simulink model "car_model"  (R2017a)
settings: Solver=VariableStepAuto  StartTime=0.0  StopTime=tf  RelTol=1e-3  AbsTol=1e-6
values from neighbouring files (symbols this model uses):
  MAX_DELTA_i = deg2rad(MAX_DELTA_i)    [run_sim.m]
  x0 = double(subs([qs0; ps0], symbs, vals))    [run_sim.m]
undefined symbols (not defined in the file or in its folder): sys
(part 1 of 2)
settings Model: Creator=brunolnetto  LastModifiedBy=brunolnetto
settings DataIOCC: SaveState=on  StateSaveName=xoutNew  OutputSaveName=youtNew

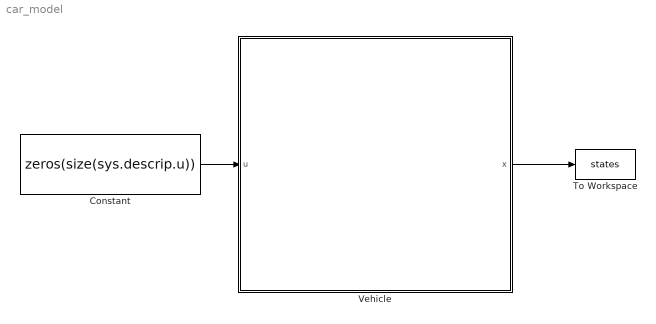
== system car_model ==
  Constant : Constant  Value=zeros(size(sys.descrip.u))
  To Workspace : ToWorkspace  VariableName=states  SaveFormat=Structure With Time  SampleTime=-1
  Vehicle : Subsystem
      mask Display: image('/home/brunolnetto/Pictures/auto_model.png');
  wires:
  Constant/1 -> Vehicle/1(u)
  Vehicle/1(x) -> To Workspace/1

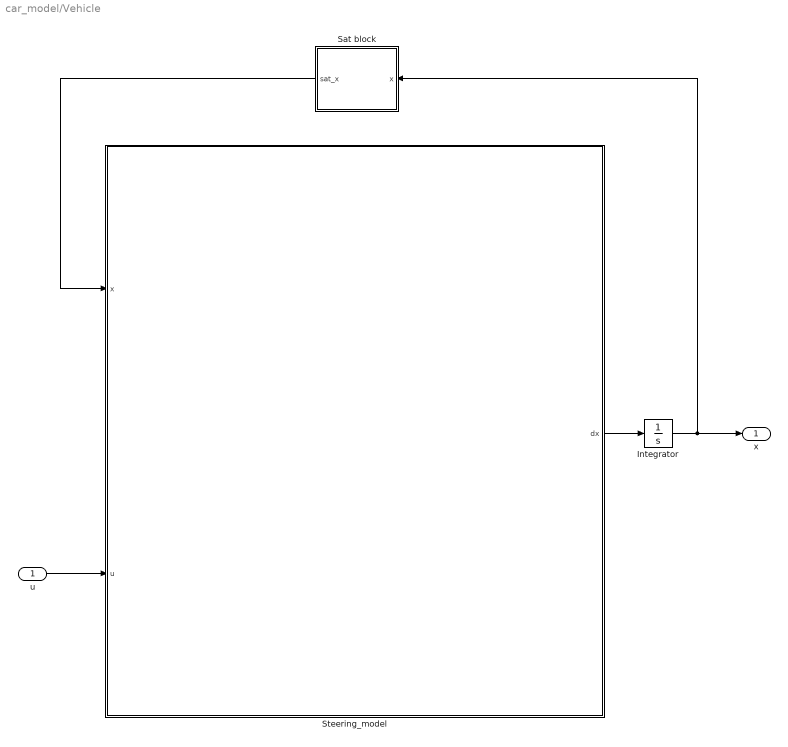
== system car_model/Vehicle ==
  u : Inport
  Integrator : Integrator  InitialCondition=x0
  Sat block : Subsystem
  Steering_model : Subsystem
      mask Display: image('/home/brunolnetto/Pictures/steer_schema.png');
  x : Outport
  wires:
  Steering_model/1(dx) -> Integrator/1
  u/1 -> Steering_model/2(u)
  Integrator/1 -> x/1, Sat block/1(x)
  Sat block/1(sat_x) -> Steering_model/1(x)

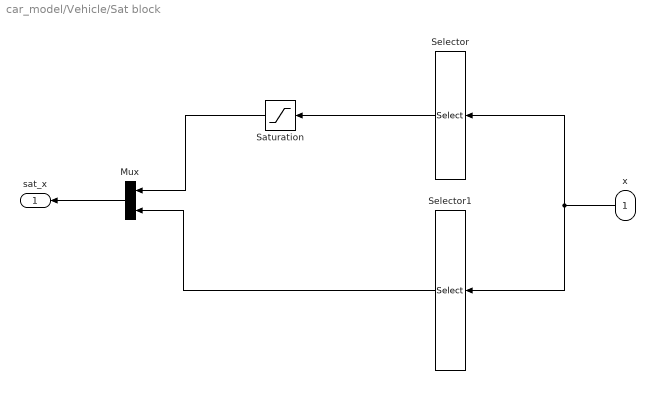
== system car_model/Vehicle/Sat block ==
  x : Inport
  Mux : Mux  Inputs=2
  Saturation : Saturate  UpperLimit=MAX_DELTA_i  LowerLimit=-MAX_DELTA_i
  Selector : Selector  InputPortWidth=13  IndexOptions=Index vector (dialog)  Indices=4  OutputSizes=1
  Selector1 : Selector  InputPortWidth=13  IndexOptions=Index vector (dialog)  Indices=[1 2. 3. 5. 6. 7. 8. 9. 10. 11. 12. 13]  OutputSizes=1
  sat_x : Outport
  wires:
  Saturation/1 -> Mux/1
  Selector/1 -> Saturation/1
  Mux/1 -> sat_x/1
  x/1 -> Selector1/1, Selector/1
  Selector1/1 -> Mux/2

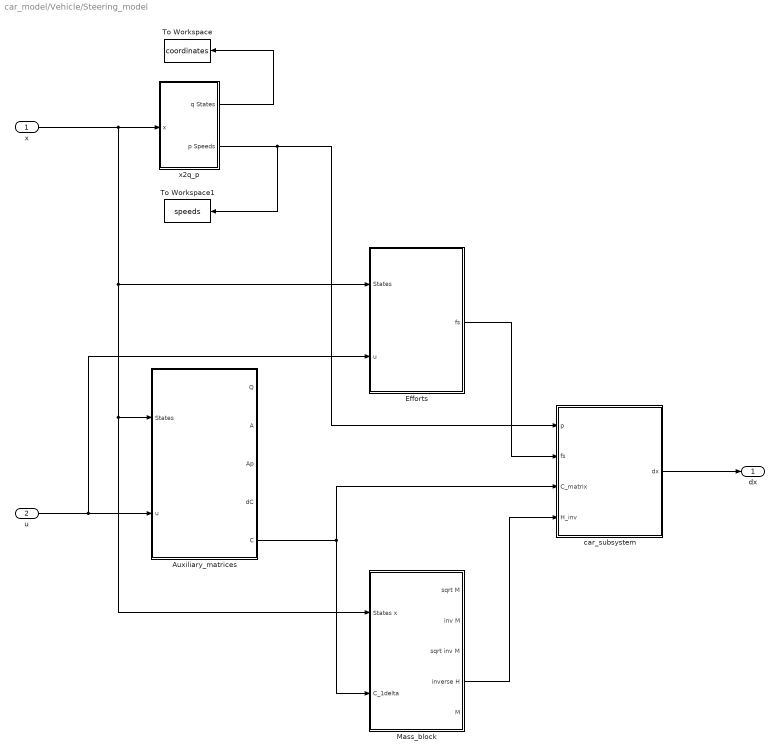
== system car_model/Vehicle/Steering_model ==
  x : Inport
  u : Inport  Port=2
  Auxiliary_matrices : Subsystem
  Efforts : Subsystem
  Mass_block : Subsystem
  To Workspace : ToWorkspace  VariableName=coordinates  SaveFormat=Structure With Time  SampleTime=-1
  To Workspace1 : ToWorkspace  VariableName=speeds  SaveFormat=Structure With Time  SampleTime=-1
  car_subsystem : Subsystem
  x2q_p : Subsystem
  dx : Outport
  wires:
  Auxiliary_matrices/5(C) -> car_subsystem/3(C_matrix), Mass_block/2("C_1delta  ")
  u/1 -> Efforts/2(u), Auxiliary_matrices/2(u)
  Mass_block/4(inverse H) -> car_subsystem/4(H_inv)
  car_subsystem/1(dx) -> dx/1
  Efforts/1(fs) -> car_subsystem/2(fs)
  x2q_p/1(q States) -> To Workspace/1
  x2q_p/2(p Speeds) -> To Workspace1/1, car_subsystem/1(p)
  x/1 -> x2q_p/1(x), Efforts/1(States), Mass_block/1(States x), Auxiliary_matrices/1(States)

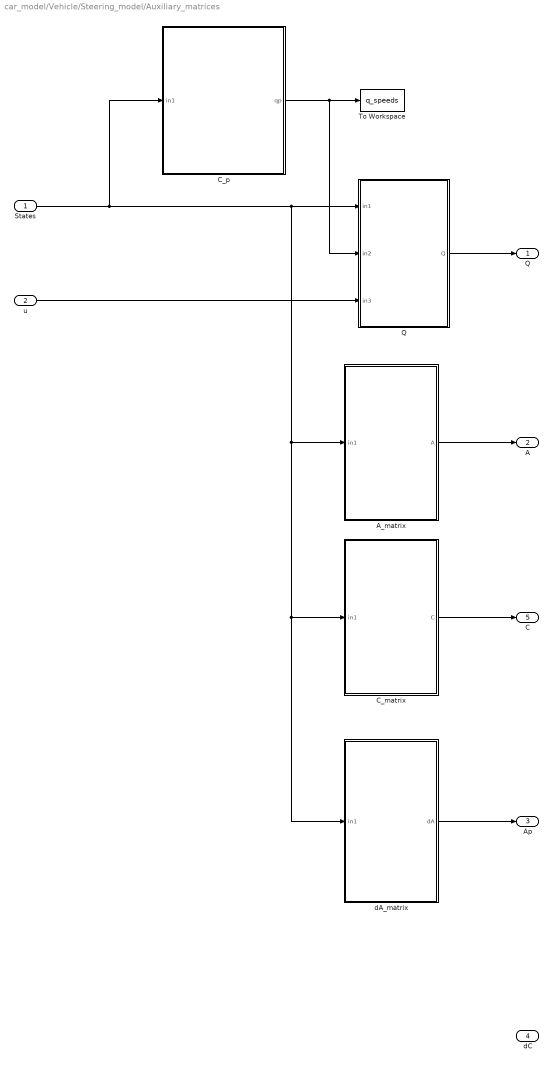
== system car_model/Vehicle/Steering_model/Auxiliary_matrices ==
  States : Inport
  u : Inport  Port=2
  A_matrix : MATLAB Function  TreatAsAtomicUnit=on
  C_matrix : MATLAB Function  TreatAsAtomicUnit=on
  C_p : MATLAB Function  TreatAsAtomicUnit=on
  Q : MATLAB Function  TreatAsAtomicUnit=on
  To Workspace : ToWorkspace  VariableName=q_speeds  SaveFormat=Structure With Time  SampleTime=-1
  dA_matrix : MATLAB Function  TreatAsAtomicUnit=on
  "Q " : Outport
  A : Outport  Port=2
  Ap : Outport  Port=3
  dC : Outport  Port=4
  C : Outport  Port=5
  wires:
  C_matrix/1(C) -> C/1
  Q/1(Q) -> "Q "/1
  A_matrix/1(A) -> A/1
  dA_matrix/1(dA) -> Ap/1
  u/1 -> Q/3(in3)
  States/1 -> C_p/1(in1), dA_matrix/1(in1), C_matrix/1(in1), A_matrix/1(in1), Q/1(in1)
  C_p/1(qp) -> To Workspace/1, Q/2(in2)

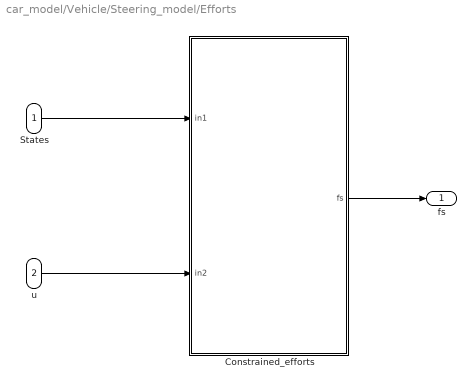
== system car_model/Vehicle/Steering_model/Efforts ==
  States : Inport
  u : Inport  Port=2
  Constrained_efforts : MATLAB Function  TreatAsAtomicUnit=on
  fs : Outport
  wires:
  States/1 -> Constrained_efforts/1(in1)
  u/1 -> Constrained_efforts/2(in2)
  Constrained_efforts/1(fs) -> fs/1

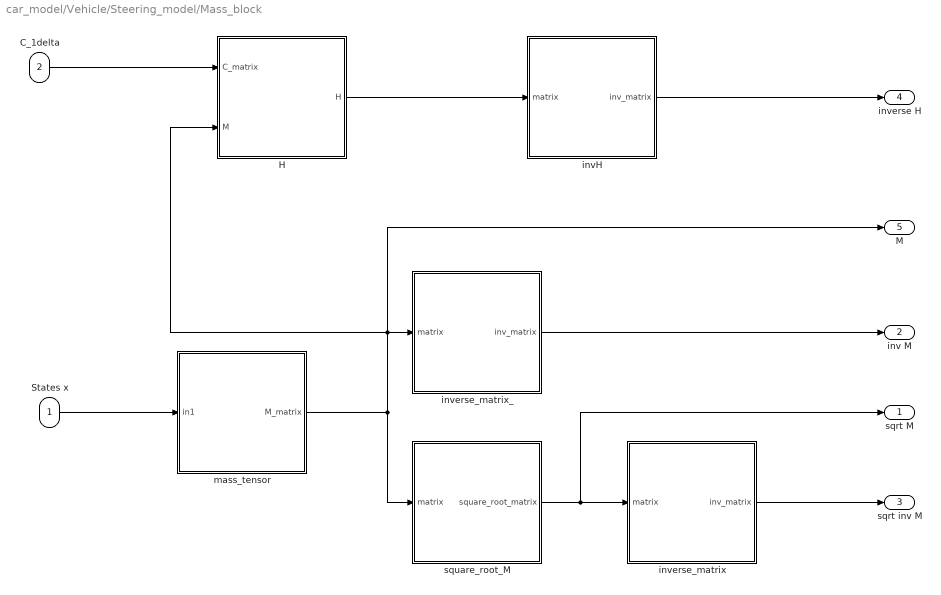
== system car_model/Vehicle/Steering_model/Mass_block ==
  States x : Inport
  "C_1delta  " : Inport  Port=2
  H : MATLAB Function  TreatAsAtomicUnit=on
  invH : MATLAB Function  TreatAsAtomicUnit=on
  inverse_matrix : MATLAB Function  TreatAsAtomicUnit=on
  inverse_matrix_ : MATLAB Function  TreatAsAtomicUnit=on
  mass_tensor : MATLAB Function  TreatAsAtomicUnit=on
  square_root_M : MATLAB Function  TreatAsAtomicUnit=on
  sqrt M : Outport
  inv M : Outport  Port=2
  sqrt inv M : Outport  Port=3
  inverse H : Outport  Port=4
  M : Outport  Port=5
  wires:
  States x/1 -> mass_tensor/1(in1)
  "C_1delta  "/1 -> H/1(C_matrix)
  inverse_matrix_/1(inv_matrix) -> inv M/1
  H/1(H) -> invH/1(matrix)
  invH/1(inv_matrix) -> inverse H/1
  inverse_matrix/1(inv_matrix) -> sqrt inv M/1
  mass_tensor/1(M_matrix) -> M/1, H/2(M), inverse_matrix_/1(matrix), square_root_M/1(matrix)
  square_root_M/1(square_root_matrix) -> sqrt M/1, inverse_matrix/1(matrix)

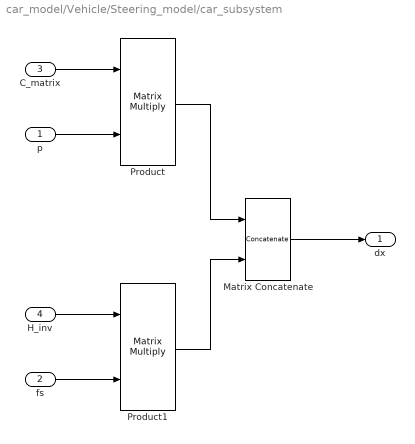
== system car_model/Vehicle/Steering_model/car_subsystem ==
  p : Inport
  fs : Inport  Port=2
  C_matrix : Inport  Port=3
  H_inv : Inport  Port=4
  Matrix Concatenate : Concatenate  ConcatenateDimension=2
  Product : Product  Multiplication=Matrix(*)
  Product1 : Product  Multiplication=Matrix(*)
  dx : Outport
  wires:
  Product/1 -> Matrix Concatenate/1
  p/1 -> Product/2
  C_matrix/1 -> Product/1
  Product1/1 -> Matrix Concatenate/2
  H_inv/1 -> Product1/1
  fs/1 -> Product1/2
  Matrix Concatenate/1 -> dx/1

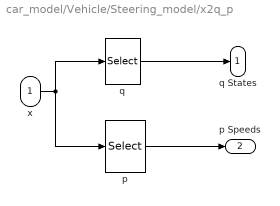
== system car_model/Vehicle/Steering_model/x2q_p ==
  x : Inport
  p : Selector  InputPortWidth=13  IndexOptions=Index vector (dialog)  Indices=[10 11 12 13]  OutputSizes=1
  q : Selector  InputPortWidth=13  IndexOptions=Index vector (dialog)  Indices=[1 2 3 4 5 6 7 8 9]  OutputSizes=1
  q States : Outport
  p Speeds : Outport  Port=2
  wires:
  x/1 -> p/1, q/1
  q/1 -> q States/1
  p/1 -> p Speeds/1

== matlab function car_model/Vehicle/Steering_model/Auxiliary_matrices/A_matrix ==
  data: in1 input; A output
function A = ConstraintMatrix(in1)

%    This function was generated by the Symbolic Math Toolbox version 7.2.

%    28-Oct-2020 21:52:18



delta_i = in1(4,:);

delta_o = in1(5,:);

theta = in1(3,:);

t2 = tan(delta_i);

t3 = tan(delta_o);

t4 = t2.*(3.0./2.0);

t5 = delta_i+theta;

t6 = cos(delta_i);

t7 = sin(t5);

t8 = cos(t5);

t9 = sin(delta_i);

A = reshape([0.0,0.0,0.0,t8,-t7,0.0,0.0,0.0,t7,t8,0.0,0.0,0.0,t6.*(-9.0./2.0)+t9.*(3.0./4.0),t6.*(3.0./4.0)+t9.*(9.0./2.0),(t3.*(3.0./2.0)-9.0./2.0).*(t2.^2+1.0).*(-2.0./9.0),0.0,0.0,0.0,0.0,(t3.^2+1.0).*(t4+9.0./2.0).*(-2.0./9.0),0.0,0.0,0.0,0.0,0.0,0.0,1.0./t6,-3.442462000000001e-1,0.0,0.0,0.0,(t4-9.0)./(cos(delta_o).*(t4+9.0)),0.0,0.0,0.0,t2.*(-1.0./3.0)-1.0,0.0,0.0,0.0,0.0,1.0,0.0,0.0,0.0],[5,9]);

end

== matlab function car_model/Vehicle/Steering_model/Mass_block/mass_tensor ==
  data: in1 input; M_matrix output
function M_matrix = Mass_matrix(in1)

%    This function was generated by the Symbolic Math Toolbox version 7.2.

%    28-Oct-2020 21:52:21



delta_i = in1(4,:);

delta_o = in1(5,:);

phi_i = in1(6,:);

phi_l = in1(9,:);

phi_o = in1(7,:);

phi_r = in1(8,:);

theta = in1(3,:);

t2 = cos(theta);

t3 = sin(theta);

t4 = cos(phi_i);

t5 = t4.^2;

t6 = cos(phi_l);

t7 = t6.^2;

t8 = cos(phi_o);

t9 = t8.^2;

t10 = cos(phi_r);

t11 = t10.^2;

t12 = t2.^2;

t13 = sin(phi_l);

t14 = t13.^2;

t15 = sin(phi_r);

t16 = t15.^2;

t17 = t3.^2;

t18 = cos(delta_i);

t19 = sin(phi_i);

t20 = t19.^2;

t21 = cos(delta_o);

t22 = sin(phi_o);

t23 = t22.^2;

t24 = t18.^2;

t25 = sin(delta_i);

t26 = t21.^2;

t27 = sin(delta_o);

t28 = t25.^2;

t29 = t20.^2;

t30 = t27.^2;

t31 = t23.^2;

t32 = phi_i.*4.0;

t33 = cos(t32);

t34 = t5.^2;

t35 = t34.*4.147690617505401e-1;

t36 = t12.*t24.*t29.*4.147690617505401e-1;

t37 = t17.*t20.*t24.*2.073845308752701e-1;

t38 = t12.*t20.*t28.*2.073845308752701e-1;

t39 = t17.*t28.*t29.*4.147690617505401e-1;

t40 = t5.*t12.*t20.*t24.*2.073845308752701e-1;

t41 = t5.*t17.*t20.*t28.*2.073845308752701e-1;

t42 = t3.*t5.*t20.*t25.*4.147690617505401e-1;

t43 = t2.*t3.*t18.*t20.*t25.*4.147690617505401e-1;

t44 = phi_o.*4.0;

t45 = cos(t44);

t46 = t9.^2;

t47 = t46.*4.147690617505401e-1;

t48 = t12.*t26.*t31.*4.147690617505401e-1;

t49 = t17.*t23.*t26.*2.073845308752701e-1;

t50 = t12.*t23.*t30.*2.073845308752701e-1;

t51 = t17.*t30.*t31.*4.147690617505401e-1;

t52 = t9.*t12.*t23.*t26.*2.073845308752701e-1;

t53 = t9.*t17.*t23.*t30.*2.073845308752701e-1;

t54 = t3.*t9.*t23.*t27.*4.147690617505401e-1;

t55 = t2.*t3.*t21.*t23.*t27.*4.147690617505401e-1;

t56 = delta_i.*2.0;

t57 = theta.*2.0;

t58 = phi_i.*3.0;

t59 = sin(t58);

t60 = cos(t56);

t61 = sin(t57);

t62 = sin(t56);

t63 = cos(t57);

t64 = delta_o.*2.0;

t65 = phi_o.*3.0;

t66 = sin(t65);

t67 = cos(t64);

t68 = sin(t64);

t70 = t33.*2.592306635940876e-2;

t71 = t2.*t5.*t18.*t20.*4.147690617505401e-1;

t72 = t2.*t3.*t18.*t25.*t29.*8.295381235010802e-1;

t73 = t2.*t3.*t5.*t18.*t20.*t25.*4.147690617505401e-1;

t69 = t35+t36+t37+t38+t39+t40+t41+t42+t43-t70-t71-t72-t73+2.592306635940876e-2;

t74 = t59.*t60.*t61.*2.592306635940876e-2;

t75 = t59.*t62.*t63.*2.592306635940876e-2;

t76 = t3.*t18.*t59.*5.184613271881752e-2;

t77 = t2.*t25.*t59.*5.184613271881752e-2;

t78 = t3.*t18.*t19.*5.184613271881752e-2;

t79 = t2.*t19.*t25.*5.184613271881752e-2;

t93 = t19.*t60.*t61.*7.776919907822627e-2;

t94 = t19.*t62.*t63.*7.776919907822627e-2;

t80 = t74+t75+t76+t77+t78+t79-t93-t94;

t82 = t45.*2.592306635940876e-2;

t83 = t2.*t9.*t21.*t23.*4.147690617505401e-1;

t84 = t2.*t3.*t21.*t27.*t31.*8.295381235010802e-1;

t85 = t2.*t3.*t9.*t21.*t23.*t27.*4.147690617505401e-1;

t81 = t47+t48+t49+t50+t51+t52+t53+t54+t55-t82-t83-t84-t85+2.592306635940876e-2;

t86 = t61.*t66.*t67.*2.592306635940876e-2;

t87 = t63.*t66.*t68.*2.592306635940876e-2;

t88 = t3.*t21.*t66.*5.184613271881752e-2;

t89 = t2.*t27.*t66.*5.184613271881752e-2;

t90 = t3.*t21.*t22.*5.184613271881752e-2;

t91 = t2.*t22.*t27.*5.184613271881752e-2;

t95 = t22.*t61.*t67.*7.776919907822627e-2;

t96 = t22.*t63.*t68.*7.776919907822627e-2;

t92 = t86+t87+t88+t89+t90+t91-t95-t96;

t97 = t2.*t3.*t15.*2.073845308752701e-1;

t98 = t3.*t11.*t15.*2.073845308752701e-1;

t99 = t97+t98-t2.*t3.*t11.*t15.*2.073845308752701e-1-t2.*t3.*t15.*t16.*4.147690617505401e-1;

t100 = t2.*t3.*t13.*2.073845308752701e-1;

t101 = t3.*t7.*t13.*2.073845308752701e-1;

t102 = t100+t101-t2.*t3.*t7.*t13.*2.073845308752701e-1-t2.*t3.*t13.*t14.*4.147690617505401e-1;

t103 = t12.*2.073845308752701e-1;

M_matrix = reshape([1.885e3,0.0,t2.*(-4.24125e3),0.0,0.0,0.0,0.0,0.0,0.0,0.0,1.885e3,t3.*(-4.24125e3),0.0,0.0,0.0,0.0,0.0,0.0,t2.*(-4.24125e3),t3.*(-4.24125e3),t12.*9.7003125e3+t17.*9.7003125e3-t33.*2.592306635940876e-2+t35+t36+t37+t38+t39+t40+t41+t42+t43-t45.*2.592306635940876e-2+t47+t48+t49+t50+t51+t52+t53+t54+t55-cos(phi_l.*4.0).*2.592306635940876e-2-cos(phi_r.*4.0).*2.592306635940876e-2+t14.*t17.*2.073845308752701e-1+t16.*t17.*2.073845308752701e-1+t12.*t14.^2.*4.147690617505401e-1+t12.*t16.^2.*4.147690617505401e-1+t7.^2.*4.147690617505401e-1+t11.^2.*4.147690617505401e-1+t2.*t7.*(t7-1.0).*4.147690617505401e-1+t2.*t11.*(t11-1.0).*4.147690617505401e-1+t7.*t12.*t14.*2.073845308752701e-1+t11.*t12.*t16.*2.073845308752701e-1-t2.*t5.*t18.*t20.*4.147690617505401e-1-t2.*t9.*t21.*t23.*4.147690617505401e-1-t2.*t3.*t18.*t25.*t29.*8.295381235010802e-1-t2.*t3.*t21.*t27.*t31.*8.295381235010802e-1-t2.*t3.*t5.*t18.*t20.*t25.*4.147690617505401e-1-t2.*t3.*t9.*t21.*t23.*t27.*4.147690617505401e-1+3.481978692265438e3,t69,t81,t80,t92,t99,t102,0.0,0.0,t69,t69,0.0,t80,0.0,0.0,0.0,0.0,0.0,t81,0.0,t81,0.0,t92,0.0,0.0,0.0,0.0,t80,t80,0.0,t5.*(-1.03692265437635e-1)-t60.*t63.*1.03692265437635e-1+t61.*t62.*1.03692265437635e-1+t5.*t60.*t63.*1.03692265437635e-1-t5.*t61.*t62.*1.03692265437635e-1+3.110767963129051e-1,0.0,0.0,0.0,0.0,0.0,t92,0.0,t92,0.0,t9.*(-1.03692265437635e-1)+t61.*t68.*1.03692265437635e-1-t63.*t67.*1.03692265437635e-1-t9.*t61.*t68.*1.03692265437635e-1+t9.*t63.*t67.*1.03692265437635e-1+3.110767963129051e-1,0.0,0.0,0.0,0.0,t99,0.0,0.0,0.0,0.0,t103+t11.*t17.*2.073845308752701e-1+t16.*t17.*4.147690617505401e-1,0.0,0.0,0.0,t102,0.0,0.0,0.0,0.0,0.0,t103+t7.*t17.*2.073845308752701e-1+t14.*t17.*4.147690617505401e-1],[9,9]);

end

== matlab function car_model/Vehicle/Steering_model/Auxiliary_matrices/C_matrix ==
  data: in1 input; C output
function C = KinematicMatrix(in1)

%    This function was generated by the Symbolic Math Toolbox version 7.2.

%    28-Oct-2020 21:52:18



delta_i = in1(4,:);

delta_o = in1(5,:);

theta = in1(3,:);

t2 = cos(delta_i);

t3 = cos(theta);

t4 = t3.*(9.0./2.0);

t5 = sin(theta);

t6 = t5.*(3.0./4.0);

t7 = delta_i.*2.0;

t8 = t7+theta;

t9 = cos(delta_o);

t10 = 1.0./t9;

t11 = t2.*9.0;

t12 = sin(delta_i);

t13 = t12.*(3.0./2.0);

t14 = t11+t13;

t15 = 1.0./t14;

t16 = sin(t8);

t17 = t5.*(9.0./2.0);

t18 = cos(t8);

t19 = delta_o.*2.0;

C = reshape([t4+t6,t3.*(-3.0./4.0)+t17,1.0,0.0,0.0,0.0,0.0,0.0,0.0,0.0,0.0,0.0,(cos(t7).*(9.0./2.0)+sin(t7).*(3.0./2.0)+9.0./2.0)./(cos(t19).*(9.0./2.0)-sin(t19).*(3.0./2.0)+9.0./2.0),1.0,0.0,0.0,0.0,0.0,t2.*t10.*t15.*(t4+t6-t16.*(3.0./4.0)+t18.*(9.0./2.0)).*3.442462000000001e-1,t2.*t10.*t15.*(t3.*(-3.0./4.0)+t16.*(9.0./2.0)+t17+t18.*(3.0./4.0)).*3.442462000000001e-1,0.0,0.0,0.0,t2.*t10.*t15.*(t11-t13),1.0,0.0,0.0,0.0,0.0,0.0,0.0,0.0,0.0,0.0,(9.0./2.0)./(tan(delta_i).*(3.0./2.0)+9.0./2.0),1.0],[9,4]);

end

== matlab function car_model/Vehicle/Steering_model/Auxiliary_matrices/Q ==
  data: in1 input; in2 input; in3 input; Q output
function Q = EffortVector(in1,in2,in3)

%    This function was generated by the Symbolic Math Toolbox version 7.2.

%    28-Oct-2020 21:52:17



delta_i = in1(4,:);

delta_o = in1(5,:);

deltap_i = in2(4,:);

deltap_o = in2(5,:);

f_phi_i = in3(1,:);

f_phi_l = in3(4,:);

f_phi_o = in3(2,:);

f_phi_r = in3(3,:);

phi_i = in1(6,:);

phi_l = in1(9,:);

phi_o = in1(7,:);

phi_r = in1(8,:);

phip_i = in2(6,:);

phip_l = in2(9,:);

phip_o = in2(7,:);

phip_r = in2(8,:);

thetap = in2(3,:);

theta = in1(3,:);

t2 = thetap.^2;

t3 = theta.*2.0;

t4 = sin(theta);

t5 = phip_l.^2;

t6 = phip_r.^2;

t7 = phip_i.^2;

t8 = phip_o.^2;

t9 = delta_i.*2.0;

t10 = deltap_i.^2;

t11 = delta_o.*2.0;

t12 = deltap_o.^2;

t13 = phi_i.*2.0;

t14 = t3+t9+t13;

t15 = sin(t14);

t16 = phi_o.*2.0;

t17 = t3+t11+t16;

t18 = sin(t17);

t19 = t3+t9-t13;

t20 = sin(t19);

t21 = phi_i.*4.0;

t22 = t3+t9+t21;

t23 = sin(t22);

t24 = t3+t11-t16;

t25 = sin(t24);

t26 = phi_o.*4.0;

t27 = t3+t11+t26;

t28 = sin(t27);

t29 = sin(t3);

t30 = t3+t9;

t31 = sin(t30);

t32 = t3+t11;

t33 = sin(t32);

t34 = phi_l.*2.0;

t35 = phi_l.*3.0;

t36 = phi_r.*2.0;

t37 = phi_r.*3.0;

t38 = -t3+t34;

t39 = sin(t38);

t40 = t3+t34;

t41 = sin(t40);

t42 = phi_l.*4.0;

t43 = -t3+t36;

t44 = sin(t43);

t45 = t3+t36;

t46 = sin(t45);

t47 = phi_r.*4.0;

t48 = phi_i.*3.0;

t49 = phi_o.*3.0;

t50 = delta_i-t21+theta;

t51 = sin(t50);

t52 = delta_i+t21+theta;

t53 = sin(t52);

t54 = delta_o-t26+theta;

t55 = sin(t54);

t56 = delta_o+t26+theta;

t57 = sin(t56);

t58 = delta_i+theta;

t59 = sin(t58);

t60 = delta_o+theta;

t61 = sin(t60);

t62 = t42+theta;

t63 = sin(t62);

t64 = t47+theta;

t65 = sin(t64);

t66 = t3+t9-t21;

t67 = sin(t66);

t68 = t3+t11-t26;

t69 = sin(t68);

t70 = sin(t13);

t71 = sin(t21);

t72 = sin(t16);

t73 = sin(t26);

t74 = t42-theta;

t75 = sin(t74);

t76 = -t3+t42;

t77 = sin(t76);

t78 = t3+t42;

t79 = sin(t78);

t80 = t47-theta;

t81 = sin(t80);

t82 = -t3+t47;

t83 = sin(t82);

t84 = t3+t47;

t85 = sin(t84);

t86 = phi_i+t3+t9;

t87 = sin(t86);

t88 = t7.*t87.*3.888459953911314e-2;

t89 = delta_i+phi_i+theta;

t90 = sin(t89);

t91 = t10.*t23.*6.480766589852189e-3;

t92 = -phi_i+t3+t9;

t93 = sin(t92);

t94 = t7.*t93.*3.888459953911314e-2;

t95 = t3+t9+t48;

t96 = sin(t95);

t97 = t2.*t67.*6.480766589852189e-3;

t98 = t2.*t23.*6.480766589852189e-3;

t99 = t10.*t31.*3.888459953911314e-2;

t100 = t7.*t31.*5.184613271881752e-2;

t101 = t2.*t31.*3.888459953911314e-2;

t102 = t10.*t51.*1.296153317970438e-2;

t103 = t10.*t53.*1.296153317970438e-2;

t104 = delta_i-phi_i+theta;

t105 = sin(t104);

t106 = delta_i-t48+theta;

t107 = sin(t106);

t108 = delta_i+t48+theta;

t109 = sin(t108);

t110 = t2.*t51.*1.296153317970438e-2;

t111 = t2.*t53.*1.296153317970438e-2;

t112 = deltap_i.*phip_i.*t20.*5.184613271881752e-2;

t113 = deltap_i.*phip_i.*t23.*2.592306635940876e-2;

t114 = deltap_i.*t67.*thetap.*1.296153317970438e-2;

t115 = deltap_i.*t23.*thetap.*1.296153317970438e-2;

t116 = deltap_i.*phip_i.*t70.*1.03692265437635e-1;

t117 = deltap_i.*phip_i.*t71.*1.555383981564525e-1;

t118 = phip_i.*t20.*thetap.*5.184613271881752e-2;

t119 = phip_i.*t23.*thetap.*2.592306635940876e-2;

t120 = phip_i.*t70.*thetap.*1.03692265437635e-1;

t121 = phip_i.*t71.*thetap.*1.555383981564525e-1;

t122 = deltap_i.*t31.*thetap.*7.776919907822627e-2;

t123 = deltap_i.*phip_i.*t53.*1.03692265437635e-1;

t124 = deltap_i.*t51.*thetap.*2.592306635940876e-2;

t125 = deltap_i.*t53.*thetap.*2.592306635940876e-2;

t126 = phip_i.*t53.*thetap.*1.03692265437635e-1;

t127 = phi_o+t3+t11;

t128 = sin(t127);

t129 = t8.*t128.*3.888459953911314e-2;

t130 = delta_o+phi_o+theta;

t131 = sin(t130);

t132 = t12.*t28.*6.480766589852189e-3;

t133 = -phi_o+t3+t11;

t134 = sin(t133);

t135 = t8.*t134.*3.888459953911314e-2;

t136 = t3+t11+t49;

t137 = sin(t136);

t138 = t2.*t69.*6.480766589852189e-3;

t139 = t2.*t28.*6.480766589852189e-3;

t140 = t12.*t33.*3.888459953911314e-2;

t141 = t8.*t33.*5.184613271881752e-2;

t142 = t2.*t33.*3.888459953911314e-2;

t143 = t12.*t55.*1.296153317970438e-2;

t144 = t12.*t57.*1.296153317970438e-2;

t145 = delta_o-phi_o+theta;

t146 = sin(t145);

t147 = delta_o-t49+theta;

t148 = sin(t147);

t149 = delta_o+t49+theta;

t150 = sin(t149);

t151 = t2.*t55.*1.296153317970438e-2;

t152 = t2.*t57.*1.296153317970438e-2;

t153 = deltap_o.*phip_o.*t25.*5.184613271881752e-2;

t154 = deltap_o.*phip_o.*t28.*2.592306635940876e-2;

t155 = deltap_o.*t69.*thetap.*1.296153317970438e-2;

t156 = deltap_o.*t28.*thetap.*1.296153317970438e-2;

t157 = deltap_o.*phip_o.*t72.*1.03692265437635e-1;

t158 = deltap_o.*phip_o.*t73.*1.555383981564525e-1;

t159 = phip_o.*t25.*thetap.*5.184613271881752e-2;

t160 = phip_o.*t28.*thetap.*2.592306635940876e-2;

t161 = phip_o.*t72.*thetap.*1.03692265437635e-1;

t162 = phip_o.*t73.*thetap.*1.555383981564525e-1;

t163 = deltap_o.*t33.*thetap.*7.776919907822627e-2;

t164 = deltap_o.*phip_o.*t57.*1.03692265437635e-1;

t165 = deltap_o.*t55.*thetap.*2.592306635940876e-2;

t166 = deltap_o.*t57.*thetap.*2.592306635940876e-2;

t167 = phip_o.*t57.*thetap.*1.03692265437635e-1;

t168 = cos(theta);

t169 = cos(delta_i);

t170 = sin(t48);

t171 = sin(delta_i);

t172 = cos(t9);

t173 = cos(t3);

t174 = sin(phi_i);

t175 = sin(t9);

t176 = cos(t13);

t177 = cos(delta_o);

t178 = sin(t49);

t179 = sin(delta_o);

t180 = cos(t11);

t181 = sin(phi_o);

t182 = sin(t11);

t183 = cos(t16);

t184 = sin(phi_r);

t185 = t184.^2;

t186 = cos(phi_r);

t187 = t186.^2;

t188 = t168.^2;

t189 = t4.^2;

t190 = sin(phi_l);

t191 = t190.^2;

t192 = cos(phi_l);

t193 = t192.^2;

Q = [t2.*t4.*(-4.24125e3);t2.*t168.*4.24125e3;t88+t91+t94+t97+t98+t99+t100+t101+t102+t103+t110+t111+t112+t113+t114+t115+t116+t117+t118+t119+t120+t121+t122+t123+t124+t125+t126+t129+t132+t135+t138+t139+t140+t141+t142+t143+t144+t151+t152+t153+t154+t155+t156+t157+t158+t159+t160+t161+t162+t163+t164+t165+t166+t167-t2.*t4.*5.184613271881752e-2-t2.*t15.*2.592306635940876e-2-t2.*t18.*2.592306635940876e-2-t2.*t20.*2.592306635940876e-2-t7.*t15.*2.592306635940876e-2-t10.*t15.*2.592306635940876e-2-t8.*t18.*2.592306635940876e-2-t2.*t25.*2.592306635940876e-2-t7.*t20.*2.592306635940876e-2-t12.*t18.*2.592306635940876e-2+t2.*t29.*7.776919907822627e-2-t8.*t25.*2.592306635940876e-2+t5.*t29.*5.184613271881752e-2+t6.*t29.*5.184613271881752e-2+t2.*t39.*2.592306635940876e-2-t2.*t41.*2.592306635940876e-2+t5.*t39.*2.592306635940876e-2+t2.*t44.*2.592306635940876e-2-t5.*t41.*2.592306635940876e-2-t2.*t46.*2.592306635940876e-2+t6.*t44.*2.592306635940876e-2-t6.*t46.*2.592306635940876e-2-t2.*t59.*2.592306635940876e-2-t2.*t61.*2.592306635940876e-2+t2.*t63.*1.296153317970438e-2+t2.*t65.*1.296153317970438e-2-t10.*t59.*2.592306635940876e-2-t12.*t61.*2.592306635940876e-2-t2.*t75.*1.296153317970438e-2-t2.*t77.*6.480766589852189e-3+t2.*t79.*6.480766589852189e-3-t2.*t81.*1.296153317970438e-2-t2.*t83.*6.480766589852189e-3+t2.*t85.*6.480766589852189e-3-t7.*t90.*2.592306635940876e-2-t7.*t96.*3.888459953911314e-2-t7.*t105.*2.592306635940876e-2-t7.*t107.*7.776919907822627e-2-t7.*t109.*7.776919907822627e-2-t8.*t131.*2.592306635940876e-2-t8.*t137.*3.888459953911314e-2-t8.*t146.*2.592306635940876e-2-t8.*t148.*7.776919907822627e-2-t8.*t150.*7.776919907822627e-2-t7.*sin(phi_i.*-3.0+t3+t9).*3.888459953911314e-2-t10.*sin(phi_i.*-2.0+t3+t9).*2.592306635940876e-2+t10.*sin(phi_i.*-4.0+t3+t9).*6.480766589852189e-3-t8.*sin(phi_o.*-3.0+t3+t11).*3.888459953911314e-2-t12.*sin(phi_o.*-2.0+t3+t11).*2.592306635940876e-2+t12.*sin(phi_o.*-4.0+t3+t11).*6.480766589852189e-3+t5.*sin(phi_l+t3).*3.888459953911314e-2+t6.*sin(phi_r+t3).*3.888459953911314e-2-t5.*sin(phi_l+theta).*2.592306635940876e-2-t6.*sin(phi_r+theta).*2.592306635940876e-2-t5.*sin(t3+t35).*3.888459953911314e-2-t6.*sin(t3+t37).*3.888459953911314e-2-t5.*sin(t35+theta).*7.776919907822627e-2-t6.*sin(t37+theta).*7.776919907822627e-2-t5.*sin(phi_l-t3).*3.888459953911314e-2-t6.*sin(phi_r-t3).*3.888459953911314e-2+t5.*sin(phi_l-theta).*2.592306635940876e-2+t6.*sin(phi_r-theta).*2.592306635940876e-2+t5.*sin(-t3+t35).*3.888459953911314e-2+t6.*sin(-t3+t37).*3.888459953911314e-2+t5.*sin(t35-theta).*7.776919907822627e-2+t6.*sin(t37-theta).*7.776919907822627e-2+phip_l.*thetap.*sin(t34).*1.03692265437635e-1+phip_l.*thetap.*sin(t42).*1.555383981564525e-1+phip_r.*thetap.*sin(t36).*1.03692265437635e-1+phip_r.*thetap.*sin(t47).*1.555383981564525e-1-deltap_i.*phip_i.*t15.*5.184613271881752e-2-deltap_o.*phip_o.*t18.*5.184613271881752e-2-deltap_i.*phip_i.*t51.*1.03692265437635e-1-deltap_i.*phip_i.*t67.*2.592306635940876e-2-deltap_o.*phip_o.*t55.*1.03692265437635e-1-deltap_o.*phip_o.*t69.*2.592306635940876e-2-deltap_i.*t15.*thetap.*5.184613271881752e-2-deltap_i.*t20.*thetap.*5.184613271881752e-2-deltap_o.*t18.*thetap.*5.184613271881752e-2-deltap_o.*t25.*thetap.*5.184613271881752e-2-deltap_i.*t59.*thetap.*5.184613271881752e-2-deltap_o.*t61.*thetap.*5.184613271881752e-2-phip_i.*t15.*thetap.*5.184613271881752e-2-phip_o.*t18.*thetap.*5.184613271881752e-2-phip_l.*t39.*thetap.*5.184613271881752e-2-phip_l.*t41.*thetap.*5.184613271881752e-2-phip_i.*t51.*thetap.*1.03692265437635e-1-phip_r.*t44.*thetap.*5.184613271881752e-2-phip_r.*t46.*thetap.*5.184613271881752e-2-phip_o.*t55.*thetap.*1.03692265437635e-1+phip_l.*t63.*thetap.*1.03692265437635e-1-phip_i.*t67.*thetap.*2.592306635940876e-2+phip_r.*t65.*thetap.*1.03692265437635e-1-phip_o.*t69.*thetap.*2.592306635940876e-2+phip_l.*t75.*thetap.*1.03692265437635e-1+phip_l.*t77.*thetap.*2.592306635940876e-2+phip_l.*t79.*thetap.*2.592306635940876e-2+phip_r.*t81.*thetap.*1.03692265437635e-1+phip_r.*t83.*thetap.*2.592306635940876e-2+phip_r.*t85.*thetap.*2.592306635940876e-2;t88+t91+t94+t97+t98+t99+t100+t101+t102+t103+t110+t111+t112+t113+t114+t115+t116+t117+t118+t119+t120+t121+t122+t123+t124+t125+t126-t2.*t15.*2.592306635940876e-2-t2.*t20.*2.592306635940876e-2-t7.*t15.*2.592306635940876e-2-t10.*t15.*2.592306635940876e-2-t7.*t20.*2.592306635940876e-2-t10.*t20.*2.592306635940876e-2-t2.*t59.*2.592306635940876e-2-t10.*t59.*2.592306635940876e-2+t10.*t67.*6.480766589852189e-3-t7.*t90.*2.592306635940876e-2-t7.*t96.*3.888459953911314e-2-t7.*t105.*2.592306635940876e-2-t7.*t107.*7.776919907822627e-2-t7.*t109.*7.776919907822627e-2-t7.*sin(t3+t9-t48).*3.888459953911314e-2-deltap_i.*phip_i.*t15.*5.184613271881752e-2-deltap_i.*phip_i.*t51.*1.03692265437635e-1-deltap_i.*phip_i.*t67.*2.592306635940876e-2-deltap_i.*t15.*thetap.*5.184613271881752e-2-deltap_i.*t20.*thetap.*5.184613271881752e-2-deltap_i.*t59.*thetap.*5.184613271881752e-2-phip_i.*t15.*thetap.*5.184613271881752e-2-phip_i.*t51.*thetap.*1.03692265437635e-1-phip_i.*t67.*thetap.*2.592306635940876e-2;t129+t132+t135+t138+t139+t140+t141+t142+t143+t144+t151+t152+t153+t154+t155+t156+t157+t158+t159+t160+t161+t162+t163+t164+t165+t166+t167-t2.*t18.*2.592306635940876e-2-t8.*t18.*2.592306635940876e-2-t2.*t25.*2.592306635940876e-2-t12.*t18.*2.592306635940876e-2-t8.*t25.*2.592306635940876e-2-t12.*t25.*2.592306635940876e-2-t2.*t61.*2.592306635940876e-2-t12.*t61.*2.592306635940876e-2+t12.*t69.*6.480766589852189e-3-t8.*t131.*2.592306635940876e-2-t8.*t137.*3.888459953911314e-2-t8.*t146.*2.592306635940876e-2-t8.*t148.*7.776919907822627e-2-t8.*t150.*7.776919907822627e-2-t8.*sin(t3+t11-t49).*3.888459953911314e-2-deltap_o.*phip_o.*t18.*5.184613271881752e-2-deltap_o.*phip_o.*t55.*1.03692265437635e-1-deltap_o.*phip_o.*t69.*2.592306635940876e-2-deltap_o.*t18.*thetap.*5.184613271881752e-2-deltap_o.*t25.*thetap.*5.184613271881752e-2-deltap_o.*t61.*thetap.*5.184613271881752e-2-phip_o.*t18.*thetap.*5.184613271881752e-2-phip_o.*t55.*thetap.*1.03692265437635e-1-phip_o.*t69.*thetap.*2.592306635940876e-2;f_phi_i-t2.*t70.*5.184613271881752e-2-t2.*t71.*7.776919907822627e-2-t7.*t70.*5.184613271881752e-2-t10.*t70.*5.184613271881752e-2-t10.*t71.*7.776919907822627e-2-deltap_i.*t70.*thetap.*1.03692265437635e-1-deltap_i.*t71.*thetap.*1.555383981564525e-1-deltap_i.*phip_i.*t29.*t172.*1.03692265437635e-1-deltap_i.*phip_i.*t173.*t175.*1.03692265437635e-1-phip_i.*t29.*t172.*thetap.*1.03692265437635e-1-phip_i.*t173.*t175.*thetap.*1.03692265437635e-1+t2.*t4.*t71.*t171.*1.03692265437635e-1+t4.*t10.*t71.*t171.*1.03692265437635e-1-t2.*t29.*t70.*t175.*5.184613271881752e-2+t2.*t29.*t71.*t175.*2.592306635940876e-2-t7.*t29.*t70.*t175.*5.184613271881752e-2-t10.*t29.*t70.*t175.*5.184613271881752e-2+t10.*t29.*t71.*t175.*2.592306635940876e-2+t2.*t4.*t170.*t171.*5.184613271881752e-2+t2.*t4.*t171.*t174.*5.184613271881752e-2+t4.*t10.*t170.*t171.*5.184613271881752e-2+t4.*t10.*t171.*t174.*5.184613271881752e-2+t2.*t29.*t170.*t175.*5.184613271881752e-2-t2.*t29.*t174.*t175.*1.555383981564525e-1+t10.*t29.*t170.*t175.*5.184613271881752e-2-t10.*t29.*t174.*t175.*1.555383981564525e-1-t2.*t71.*t168.*t169.*1.03692265437635e-1+t2.*t70.*t172.*t173.*5.184613271881752e-2-t2.*t71.*t172.*t173.*2.592306635940876e-2-t10.*t71.*t168.*t169.*1.03692265437635e-1+t7.*t70.*t172.*t173.*5.184613271881752e-2+t10.*t70.*t172.*t173.*5.184613271881752e-2-t10.*t71.*t172.*t173.*2.592306635940876e-2-t2.*t168.*t169.*t170.*5.184613271881752e-2-t2.*t168.*t169.*t174.*5.184613271881752e-2-t2.*t170.*t172.*t173.*5.184613271881752e-2-t10.*t168.*t169.*t170.*5.184613271881752e-2+t2.*t172.*t173.*t174.*1.555383981564525e-1-t10.*t168.*t169.*t174.*5.184613271881752e-2-t10.*t170.*t172.*t173.*5.184613271881752e-2+t10.*t172.*t173.*t174.*1.555383981564525e-1+deltap_i.*phip_i.*t29.*t172.*t176.*1.03692265437635e-1+deltap_i.*phip_i.*t173.*t175.*t176.*1.03692265437635e-1+deltap_i.*t4.*t71.*t171.*thetap.*2.073845308752701e-1-deltap_i.*t29.*t70.*t175.*thetap.*1.03692265437635e-1+deltap_i.*t29.*t71.*t175.*thetap.*5.184613271881752e-2+deltap_i.*t4.*t170.*t171.*thetap.*1.03692265437635e-1+deltap_i.*t4.*t171.*t174.*thetap.*1.03692265437635e-1+deltap_i.*t29.*t170.*t175.*thetap.*1.03692265437635e-1-deltap_i.*t29.*t174.*t175.*thetap.*3.110767963129051e-1-deltap_i.*t71.*t168.*t169.*thetap.*2.073845308752701e-1+deltap_i.*t70.*t172.*t173.*thetap.*1.03692265437635e-1-deltap_i.*t71.*t172.*t173.*thetap.*5.184613271881752e-2-deltap_i.*t168.*t169.*t170.*thetap.*1.03692265437635e-1-deltap_i.*t168.*t169.*t174.*thetap.*1.03692265437635e-1-deltap_i.*t170.*t172.*t173.*thetap.*1.03692265437635e-1+deltap_i.*t172.*t173.*t174.*thetap.*3.110767963129051e-1+phip_i.*t29.*t172.*t176.*thetap.*1.03692265437635e-1+phip_i.*t173.*t175.*t176.*thetap.*1.03692265437635e-1;f_phi_o-t2.*t72.*5.184613271881752e-2-t2.*t73.*7.776919907822627e-2-t8.*t72.*5.184613271881752e-2-t12.*t72.*5.184613271881752e-2-t12.*t73.*7.776919907822627e-2-deltap_o.*t72.*thetap.*1.03692265437635e-1-deltap_o.*t73.*thetap.*1.555383981564525e-1-deltap_o.*phip_o.*t29.*t180.*1.03692265437635e-1-deltap_o.*phip_o.*t173.*t182.*1.03692265437635e-1-phip_o.*t29.*t180.*thetap.*1.03692265437635e-1-phip_o.*t173.*t182.*thetap.*1.03692265437635e-1+t2.*t4.*t73.*t179.*1.03692265437635e-1+t4.*t12.*t73.*t179.*1.03692265437635e-1-t2.*t29.*t72.*t182.*5.184613271881752e-2+t2.*t29.*t73.*t182.*2.592306635940876e-2-t8.*t29.*t72.*t182.*5.184613271881752e-2-t12.*t29.*t72.*t182.*5.184613271881752e-2+t12.*t29.*t73.*t182.*2.592306635940876e-2+t2.*t4.*t178.*t179.*5.184613271881752e-2+t2.*t4.*t179.*t181.*5.184613271881752e-2+t4.*t12.*t178.*t179.*5.184613271881752e-2+t4.*t12.*t179.*t181.*5.184613271881752e-2+t2.*t29.*t178.*t182.*5.184613271881752e-2-t2.*t29.*t181.*t182.*1.555383981564525e-1+t12.*t29.*t178.*t182.*5.184613271881752e-2-t12.*t29.*t181.*t182.*1.555383981564525e-1-t2.*t73.*t168.*t177.*1.03692265437635e-1+t2.*t72.*t173.*t180.*5.184613271881752e-2-t2.*t73.*t173.*t180.*2.592306635940876e-2-t12.*t73.*t168.*t177.*1.03692265437635e-1+t8.*t72.*t173.*t180.*5.184613271881752e-2+t12.*t72.*t173.*t180.*5.184613271881752e-2-t12.*t73.*t173.*t180.*2.592306635940876e-2-t2.*t168.*t177.*t178.*5.184613271881752e-2-t2.*t168.*t177.*t181.*5.184613271881752e-2-t2.*t173.*t178.*t180.*5.184613271881752e-2-t12.*t168.*t177.*t178.*5.184613271881752e-2+t2.*t173.*t180.*t181.*1.555383981564525e-1-t12.*t168.*t177.*t181.*5.184613271881752e-2-t12.*t173.*t178.*t180.*5.184613271881752e-2+t12.*t173.*t180.*t181.*1.555383981564525e-1+deltap_o.*phip_o.*t29.*t180.*t183.*1.03692265437635e-1+deltap_o.*phip_o.*t173.*t182.*t183.*1.03692265437635e-1+deltap_o.*t4.*t73.*t179.*thetap.*2.073845308752701e-1-deltap_o.*t29.*t72.*t182.*thetap.*1.03692265437635e-1+deltap_o.*t29.*t73.*t182.*thetap.*5.184613271881752e-2+deltap_o.*t4.*t178.*t179.*thetap.*1.03692265437635e-1+deltap_o.*t4.*t179.*t181.*thetap.*1.03692265437635e-1+deltap_o.*t29.*t178.*t182.*thetap.*1.03692265437635e-1-deltap_o.*t29.*t181.*t182.*thetap.*3.110767963129051e-1-deltap_o.*t73.*t168.*t177.*thetap.*2.073845308752701e-1+deltap_o.*t72.*t173.*t180.*thetap.*1.03692265437635e-1-deltap_o.*t73.*t173.*t180.*thetap.*5.184613271881752e-2-deltap_o.*t168.*t177.*t178.*thetap.*1.03692265437635e-1-deltap_o.*t168.*t177.*t181.*thetap.*1.03692265437635e-1-deltap_o.*t173.*t178.*t180.*thetap.*1.03692265437635e-1+deltap_o.*t173.*t180.*t181.*thetap.*3.110767963129051e-1+phip_o.*t29.*t180.*t183.*thetap.*1.03692265437635e-1+phip_o.*t173.*t182.*t183.*thetap.*1.03692265437635e-1;f_phi_r-t2.*t184.*t188.*2.073845308752701e-1+t2.*t184.*t189.*2.073845308752701e-1+phip_r.*t4.*t168.*thetap.*4.147690617505401e-1-t2.*t168.*t184.*t187.*2.073845308752701e-1-t2.*t184.*t185.*t186.*2.073845308752701e-1+t2.*t184.*t185.*t188.*4.147690617505401e-1-t2.*t184.*t186.*t187.*6.221535926258102e-1-t2.*t184.*t185.*t189.*4.147690617505401e-1+t2.*t184.*t186.*t189.*2.073845308752701e-1+t2.*t184.*t187.*t188.*2.073845308752701e-1-t2.*t184.*t187.*t189.*2.073845308752701e-1-t6.*t184.*t186.*t189.*2.073845308752701e-1-phip_r.*t4.*t168.*t185.*thetap.*8.295381235010802e-1-phip_r.*t4.*t168.*t187.*thetap.*4.147690617505401e-1+t2.*t168.*t184.*t185.*t186.*4.147690617505401e-1-t2.*t168.*t184.*t186.*t187.*4.147690617505401e-1+t2.*t184.*t185.*t186.*t188.*6.221535926258102e-1+t2.*t184.*t186.*t187.*t188.*2.073845308752701e-1;f_phi_l-t2.*t188.*t190.*2.073845308752701e-1+t2.*t189.*t190.*2.073845308752701e-1+phip_l.*t4.*t168.*thetap.*4.147690617505401e-1-t2.*t168.*t190.*t193.*2.073845308752701e-1+t2.*t188.*t190.*t191.*4.147690617505401e-1-t2.*t189.*t190.*t191.*4.147690617505401e-1+t2.*t188.*t190.*t193.*2.073845308752701e-1+t2.*t189.*t190.*t192.*2.073845308752701e-1-t2.*t189.*t190.*t193.*2.073845308752701e-1-t2.*t190.*t191.*t192.*2.073845308752701e-1-t5.*t189.*t190.*t192.*2.073845308752701e-1-t2.*t190.*t192.*t193.*6.221535926258102e-1-phip_l.*t4.*t168.*t191.*thetap.*8.295381235010802e-1-phip_l.*t4.*t168.*t193.*thetap.*4.147690617505401e-1+t2.*t168.*t190.*t191.*t192.*4.147690617505401e-1-t2.*t168.*t190.*t192.*t193.*4.147690617505401e-1+t2.*t188.*t190.*t191.*t192.*6.221535926258102e-1+t2.*t188.*t190.*t192.*t193.*2.073845308752701e-1];

end

== matlab function car_model/Vehicle/Steering_model/Auxiliary_matrices/dA_matrix ==
  data: in1 input; dA output
function dA = dConstraintMatrix(in1)

%    This function was generated by the Symbolic Math Toolbox version 7.2.

%    28-Oct-2020 21:52:19



delta_i = in1(4,:);

delta_o = in1(5,:);

p1 = in1(10,:);

p2 = in1(11,:);

theta = in1(3,:);

t2 = tan(delta_i);

t3 = tan(delta_o);

t4 = t2.^2;

t5 = t4+1.0;

t6 = delta_i.*2.0;

t7 = delta_o.*2.0;

t8 = t3.^2;

t9 = t8+1.0;

t10 = cos(t6);

t11 = t10.*(9.0./2.0);

t12 = sin(t6);

t13 = t12.*(3.0./2.0);

t14 = t11+t13+9.0./2.0;

t15 = cos(t7);

t16 = t15.*(9.0./2.0);

t17 = sin(t7);

t20 = t17.*(3.0./2.0);

t18 = t16-t20+9.0./2.0;

t19 = 1.0./t18;

t21 = t2.*(3.0./2.0);

t22 = cos(delta_o);

t23 = 1.0./t22;

t24 = t21+9.0;

t25 = t21-9.0;

t26 = 1.0./t24;

t27 = delta_i+theta;

t28 = sin(t27);

t29 = cos(t27);

t30 = cos(delta_i);

t31 = sin(delta_i);

t32 = p1.*t29;

t33 = p2.*t14.*t19.*t29;

t34 = -p1.*t28-p2.*t14.*t19.*t28;

dA = reshape([0.0,0.0,0.0,t34,-t32-t33,0.0,0.0,0.0,t32+t33,t34,0.0,0.0,0.0,p2.*t14.*t19.*(t30.*(3.0./4.0)+t31.*(9.0./2.0)),p2.*t14.*t19.*(t30.*(9.0./2.0)-t31.*(3.0./4.0)),p2.*t5.*t9.*(-1.0./3.0)-p2.*t2.*t5.*t14.*t19.*(t3.*(3.0./2.0)-9.0./2.0).*(4.0./9.0),0.0,0.0,0.0,0.0,p2.*t3.*t9.*(t21+9.0./2.0).*(-4.0./9.0)-p2.*t5.*t9.*t14.*t19.*(1.0./3.0),0.0,0.0,0.0,0.0,0.0,0.0,p2.*t14.*t19.*1.0./t30.^2.*t31,0.0,0.0,0.0,0.0,p2.*t14.*t19.*(t5.*t23.*t26.*(3.0./2.0)-t5.*t23.*1.0./t24.^2.*t25.*(3.0./2.0))+p2.*1.0./t22.^2.*t25.*t26.*sin(delta_o),0.0,0.0,0.0,p2.*t5.*t14.*t19.*(-1.0./3.0),0.0,0.0,0.0,0.0,0.0,0.0,0.0,0.0],[5,9]);

end
